simulink model "EPT"  (R2019b)
settings: Solver=FixedStepDiscrete  StartTime=0.0  StopTime=5  FixedStep=0.005  RelTol=1e-3  EnableMultiTasking=on
PreLoadFcn:
  | try, model_open; catch, disp('Error occurred while executing model pre-load callback: model_open.m'); disp('Please assure that the MATLAB working directory is set to the model directory before opening.'); end
InitFcn:
  | try, model_open; catch, end
undefined symbols (not defined in the file or in its folder): Bridge, GCM, H, ln, raptor_get_param_eval, raptor_get_safe_string, raptor_xcp_function
libraries: Raptor_lib x2810, simulink x374, hdlsllib x19
(part 42 of 45)

== system EPT/Foreground_TimeBase_5ms/E//W /BP-OBU_E//W/BP-OBU_E//W/BP-OBU_Warning//Fault_G5/Delay41/CycleTrigger ==
  In1 : Inport
  In2 : Inport  Port=2
  Add : Sum
  Add2 : Sum  Inputs=+-
  Constant2 : Constant  Value=0
  Constant3 : Constant
  Data Type Conversion1 : DataTypeConversion
  Data Type Conversion2 : DataTypeConversion
  Relational Operator1 : RelationalOperator  OutDataTypeStr=boolean  RndMeth=Simplest
  Saturation : Saturate  UpperLimit=inf  LowerLimit=2
  Switch : Switch  Threshold=1
  Unit Delay : UnitDelay  SampleTime=-1  HasFrameUpgradeWarning=on
  Trigger : Outport  VectorParamsAs1DForOutWhenUnconnected=off
  wires:
  Constant3/1 -> Add2/2
  In2/1 -> Saturation/1
  Add2/1 -> Data Type Conversion1/1
  Data Type Conversion2/1 -> Switch/2, Add/2
  Constant2/1 -> Switch/3
  Data Type Conversion1/1 -> Relational Operator1/2
  Relational Operator1/1 -> Trigger/1
  Switch/1 -> Unit Delay/1, Relational Operator1/1
  Unit Delay/1 -> Add/1
  In1/1 -> Data Type Conversion2/1
  Add/1 -> Switch/1
  Saturation/1 -> Add2/1

== system EPT/Foreground_TimeBase_5ms/E//W /BP-OBU_E//W/BP-OBU_E//W/BP-OBU_Warning//Fault_G5/Delay42/CycleTrigger ==
  In1 : Inport
  In2 : Inport  Port=2
  Add : Sum
  Add2 : Sum  Inputs=+-
  Constant2 : Constant  Value=0
  Constant3 : Constant
  Data Type Conversion1 : DataTypeConversion
  Data Type Conversion2 : DataTypeConversion
  Relational Operator1 : RelationalOperator  OutDataTypeStr=boolean  RndMeth=Simplest
  Saturation : Saturate  UpperLimit=inf  LowerLimit=2
  Switch : Switch  Threshold=1
  Unit Delay : UnitDelay  SampleTime=-1  HasFrameUpgradeWarning=on
  Trigger : Outport  VectorParamsAs1DForOutWhenUnconnected=off
  wires:
  Saturation/1 -> Add2/1
  Add/1 -> Switch/1
  In1/1 -> Data Type Conversion2/1
  Unit Delay/1 -> Add/1
  Switch/1 -> Relational Operator1/1, Unit Delay/1
  Relational Operator1/1 -> Trigger/1
  Data Type Conversion1/1 -> Relational Operator1/2
  Constant2/1 -> Switch/3
  Data Type Conversion2/1 -> Add/2, Switch/2
  Add2/1 -> Data Type Conversion1/1
  In2/1 -> Saturation/1
  Constant3/1 -> Add2/2

== system EPT/Foreground_TimeBase_5ms/E//W /BP-OBU_E//W/BP-OBU_E//W/BP-OBU_Warning//Fault_G5/Delay43/CycleTrigger ==
  In1 : Inport
  In2 : Inport  Port=2
  Add : Sum
  Add2 : Sum  Inputs=+-
  Constant2 : Constant  Value=0
  Constant3 : Constant
  Data Type Conversion1 : DataTypeConversion
  Data Type Conversion2 : DataTypeConversion
  Relational Operator1 : RelationalOperator  OutDataTypeStr=boolean  RndMeth=Simplest
  Saturation : Saturate  UpperLimit=inf  LowerLimit=2
  Switch : Switch  Threshold=1
  Unit Delay : UnitDelay  SampleTime=-1  HasFrameUpgradeWarning=on
  Trigger : Outport  VectorParamsAs1DForOutWhenUnconnected=off
  wires:
  Constant3/1 -> Add2/2
  In2/1 -> Saturation/1
  Add2/1 -> Data Type Conversion1/1
  Data Type Conversion2/1 -> Switch/2, Add/2
  Constant2/1 -> Switch/3
  Data Type Conversion1/1 -> Relational Operator1/2
  Relational Operator1/1 -> Trigger/1
  Switch/1 -> Unit Delay/1, Relational Operator1/1
  Unit Delay/1 -> Add/1
  In1/1 -> Data Type Conversion2/1
  Add/1 -> Switch/1
  Saturation/1 -> Add2/1

== system EPT/Foreground_TimeBase_5ms/E//W /BP-OBU_E//W/BP-OBU_E//W/BP-OBU_Warning//Fault_G5/Delay44/CycleTrigger ==
  In1 : Inport
  In2 : Inport  Port=2
  Add : Sum
  Add2 : Sum  Inputs=+-
  Constant2 : Constant  Value=0
  Constant3 : Constant
  Data Type Conversion1 : DataTypeConversion
  Data Type Conversion2 : DataTypeConversion
  Relational Operator1 : RelationalOperator  OutDataTypeStr=boolean  RndMeth=Simplest
  Saturation : Saturate  UpperLimit=inf  LowerLimit=2
  Switch : Switch  Threshold=1
  Unit Delay : UnitDelay  SampleTime=-1  HasFrameUpgradeWarning=on
  Trigger : Outport  VectorParamsAs1DForOutWhenUnconnected=off
  wires:
  Saturation/1 -> Add2/1
  Add/1 -> Switch/1
  In1/1 -> Data Type Conversion2/1
  Unit Delay/1 -> Add/1
  Switch/1 -> Relational Operator1/1, Unit Delay/1
  Relational Operator1/1 -> Trigger/1
  Data Type Conversion1/1 -> Relational Operator1/2
  Constant2/1 -> Switch/3
  Data Type Conversion2/1 -> Add/2, Switch/2
  Add2/1 -> Data Type Conversion1/1
  In2/1 -> Saturation/1
  Constant3/1 -> Add2/2

== system EPT/Foreground_TimeBase_5ms/E//W /CAN_E//W/CAN_Fault/BCU CAN Fault/BCU LifeCycle Fault/If Action Subsystem10 ==
  LifeCycle : Inport
  CanWork : Inport  Port=2
  Enable : EnablePort
  Add Constant : Bias  Bias=1
  Constant1 : Constant  Value=5
  Delay1 : Delay  DelayLength=1  InitialCondition=0
  Detect Change : simulink/Logic and Bit Operations/Detect Change  vinit=0  OutDataTypeStr=boolean
  Logical Operator : Logic  AllPortsSameDT=off  OutDataTypeStr=boolean
  NOT : Logic  Operator=NOT  IconShape=distinctive  AllPortsSameDT=off  OutDataTypeStr=boolean
  NOT1 : Logic  Operator=NOT  IconShape=distinctive  AllPortsSameDT=off  OutDataTypeStr=boolean
  Relational Operator : RelationalOperator  Operator=>  OutDataTypeStr=boolean  RndMeth=Simplest
  Switch1 : Switch  Criteria=u2 > Threshold
  Switch4 : Switch  Criteria=u2 > Threshold
  initTimeFlag : Subsystem
  Trigger : Outport  VectorParamsAs1DForOutWhenUnconnected=off
  wires:
  NOT/1 -> Logical Operator/1
  Constant1/1 -> Relational Operator/2
  CanWork/1 -> NOT1/1, Logical Operator/2
  Detect Change/1 -> NOT/1
  Delay1/1 -> Add Constant/1
  Logical Operator/1 -> Switch4/2
  Relational Operator/1 -> Trigger/1
  Add Constant/1 -> Switch4/1
  Switch4/1 -> Switch1/3
  Switch1/1 -> Delay1/1, Relational Operator/1
  LifeCycle/1 -> Detect Change/1
  NOT1/1 -> Switch1/2

== system EPT/Foreground_TimeBase_5ms/E//W /CAN_E//W/CAN_Fault/BCU CAN Fault/BCU LifeCycle Fault/If Action Subsystem11 ==
  LifeCycle : Inport
  CanWork : Inport  Port=2
  Enable : EnablePort
  Add Constant : Bias  Bias=1
  Constant1 : Constant  Value=5
  Delay1 : Delay  DelayLength=1  InitialCondition=0
  Detect Change : simulink/Logic and Bit Operations/Detect Change  vinit=0  OutDataTypeStr=boolean
  Logical Operator : Logic  AllPortsSameDT=off  OutDataTypeStr=boolean
  NOT : Logic  Operator=NOT  IconShape=distinctive  AllPortsSameDT=off  OutDataTypeStr=boolean
  NOT1 : Logic  Operator=NOT  IconShape=distinctive  AllPortsSameDT=off  OutDataTypeStr=boolean
  Relational Operator : RelationalOperator  Operator=>  OutDataTypeStr=boolean  RndMeth=Simplest
  Switch1 : Switch  Criteria=u2 > Threshold
  Switch4 : Switch  Criteria=u2 > Threshold
  initTimeFlag : Subsystem
  Trigger : Outport  VectorParamsAs1DForOutWhenUnconnected=off
  wires:
  NOT/1 -> Logical Operator/1
  Constant1/1 -> Relational Operator/2
  CanWork/1 -> NOT1/1, Logical Operator/2
  Detect Change/1 -> NOT/1
  Delay1/1 -> Add Constant/1
  Logical Operator/1 -> Switch4/2
  Relational Operator/1 -> Trigger/1
  Add Constant/1 -> Switch4/1
  Switch4/1 -> Switch1/3
  Switch1/1 -> Delay1/1, Relational Operator/1
  LifeCycle/1 -> Detect Change/1
  NOT1/1 -> Switch1/2

== system EPT/Foreground_TimeBase_5ms/E//W /CAN_E//W/CAN_Fault/BCU CAN Fault/BCU LifeCycle Fault/If Action Subsystem12 ==
  LifeCycle : Inport
  CanWork : Inport  Port=2
  Enable : EnablePort
  Add Constant : Bias  Bias=1
  Constant1 : Constant  Value=5
  Delay1 : Delay  DelayLength=1  InitialCondition=0
  Detect Change : simulink/Logic and Bit Operations/Detect Change  vinit=0  OutDataTypeStr=boolean
  Logical Operator : Logic  AllPortsSameDT=off  OutDataTypeStr=boolean
  NOT : Logic  Operator=NOT  IconShape=distinctive  AllPortsSameDT=off  OutDataTypeStr=boolean
  NOT1 : Logic  Operator=NOT  IconShape=distinctive  AllPortsSameDT=off  OutDataTypeStr=boolean
  Relational Operator : RelationalOperator  Operator=>  OutDataTypeStr=boolean  RndMeth=Simplest
  Switch1 : Switch  Criteria=u2 > Threshold
  Switch4 : Switch  Criteria=u2 > Threshold
  initTimeFlag : Subsystem
  Trigger : Outport  VectorParamsAs1DForOutWhenUnconnected=off
  wires:
  NOT/1 -> Logical Operator/1
  Constant1/1 -> Relational Operator/2
  CanWork/1 -> NOT1/1, Logical Operator/2
  Detect Change/1 -> NOT/1
  Delay1/1 -> Add Constant/1
  Logical Operator/1 -> Switch4/2
  Relational Operator/1 -> Trigger/1
  Add Constant/1 -> Switch4/1
  Switch4/1 -> Switch1/3
  Switch1/1 -> Delay1/1, Relational Operator/1
  LifeCycle/1 -> Detect Change/1
  NOT1/1 -> Switch1/2

== system EPT/Foreground_TimeBase_5ms/E//W /CAN_E//W/CAN_Fault/BCU CAN Fault/BCU LifeCycle Fault/If Action Subsystem13 ==
  LifeCycle : Inport
  CanWork : Inport  Port=2
  Enable : EnablePort
  Add Constant : Bias  Bias=1
  Constant1 : Constant  Value=5
  Delay1 : Delay  DelayLength=1  InitialCondition=0
  Detect Change : simulink/Logic and Bit Operations/Detect Change  vinit=0  OutDataTypeStr=boolean
  Logical Operator : Logic  AllPortsSameDT=off  OutDataTypeStr=boolean
  NOT : Logic  Operator=NOT  IconShape=distinctive  AllPortsSameDT=off  OutDataTypeStr=boolean
  NOT1 : Logic  Operator=NOT  IconShape=distinctive  AllPortsSameDT=off  OutDataTypeStr=boolean
  Relational Operator : RelationalOperator  Operator=>  OutDataTypeStr=boolean  RndMeth=Simplest
  Switch1 : Switch  Criteria=u2 > Threshold
  Switch4 : Switch  Criteria=u2 > Threshold
  initTimeFlag : Subsystem
  Trigger : Outport  VectorParamsAs1DForOutWhenUnconnected=off
  wires:
  NOT1/1 -> Switch1/2
  LifeCycle/1 -> Detect Change/1
  Switch1/1 -> Relational Operator/1, Delay1/1
  Switch4/1 -> Switch1/3
  Add Constant/1 -> Switch4/1
  Relational Operator/1 -> Trigger/1
  Logical Operator/1 -> Switch4/2
  Delay1/1 -> Add Constant/1
  Detect Change/1 -> NOT/1
  CanWork/1 -> Logical Operator/2, NOT1/1
  Constant1/1 -> Relational Operator/2
  NOT/1 -> Logical Operator/1

== system EPT/Foreground_TimeBase_5ms/E//W /CAN_E//W/CAN_Fault/BCU CAN Fault/BCU LifeCycle Fault/If Action Subsystem18 ==
  LifeCycle : Inport
  CanWork : Inport  Port=2
  Enable : EnablePort
  Add Constant : Bias  Bias=1
  Constant1 : Constant  Value=5
  Delay1 : Delay  DelayLength=1  InitialCondition=0
  Detect Change : simulink/Logic and Bit Operations/Detect Change  vinit=0  OutDataTypeStr=boolean
  Logical Operator : Logic  AllPortsSameDT=off  OutDataTypeStr=boolean
  NOT : Logic  Operator=NOT  IconShape=distinctive  AllPortsSameDT=off  OutDataTypeStr=boolean
  NOT1 : Logic  Operator=NOT  IconShape=distinctive  AllPortsSameDT=off  OutDataTypeStr=boolean
  Relational Operator : RelationalOperator  Operator=>  OutDataTypeStr=boolean  RndMeth=Simplest
  Switch1 : Switch  Criteria=u2 > Threshold
  Switch4 : Switch  Criteria=u2 > Threshold
  initTimeFlag : Subsystem
  Trigger : Outport  VectorParamsAs1DForOutWhenUnconnected=off
  wires:
  NOT1/1 -> Switch1/2
  LifeCycle/1 -> Detect Change/1
  Switch1/1 -> Relational Operator/1, Delay1/1
  Switch4/1 -> Switch1/3
  Add Constant/1 -> Switch4/1
  Relational Operator/1 -> Trigger/1
  Logical Operator/1 -> Switch4/2
  Delay1/1 -> Add Constant/1
  Detect Change/1 -> NOT/1
  CanWork/1 -> Logical Operator/2, NOT1/1
  Constant1/1 -> Relational Operator/2
  NOT/1 -> Logical Operator/1

== system EPT/Foreground_TimeBase_5ms/E//W /CAN_E//W/CAN_Fault/BCU CAN Fault/BCU LifeCycle Fault/If Action Subsystem9 ==
  LifeCycle : Inport
  CanWork : Inport  Port=2
  Enable : EnablePort
  Add Constant : Bias  Bias=1
  Constant1 : Constant  Value=5
  Delay1 : Delay  DelayLength=1  InitialCondition=0
  Detect Change : simulink/Logic and Bit Operations/Detect Change  vinit=0  OutDataTypeStr=boolean
  Logical Operator : Logic  AllPortsSameDT=off  OutDataTypeStr=boolean
  NOT : Logic  Operator=NOT  IconShape=distinctive  AllPortsSameDT=off  OutDataTypeStr=boolean
  NOT1 : Logic  Operator=NOT  IconShape=distinctive  AllPortsSameDT=off  OutDataTypeStr=boolean
  Relational Operator : RelationalOperator  Operator=>  OutDataTypeStr=boolean  RndMeth=Simplest
  Switch1 : Switch  Criteria=u2 > Threshold
  Switch4 : Switch  Criteria=u2 > Threshold
  initTimeFlag : Subsystem
  Trigger : Outport  VectorParamsAs1DForOutWhenUnconnected=off
  wires:
  NOT/1 -> Logical Operator/1
  Constant1/1 -> Relational Operator/2
  CanWork/1 -> NOT1/1, Logical Operator/2
  Detect Change/1 -> NOT/1
  Delay1/1 -> Add Constant/1
  Logical Operator/1 -> Switch4/2
  Relational Operator/1 -> Trigger/1
  Add Constant/1 -> Switch4/1
  Switch4/1 -> Switch1/3
  Switch1/1 -> Delay1/1, Relational Operator/1
  LifeCycle/1 -> Detect Change/1
  NOT1/1 -> Switch1/2

== system EPT/Foreground_TimeBase_5ms/E//W /CAN_E//W/CAN_Fault/BCU CAN Fault/BCU LifeCycle Fault/Latch10 ==
  Latch : Inport
  Reset : Inport  Port=2
  Switch1 : Switch  Criteria=u2 > Threshold
  Switch3 : Switch  Criteria=u2 > Threshold
  Unit Delay1 : UnitDelay  SampleTime=-1  HasFrameUpgradeWarning=on
  Output : Outport  VectorParamsAs1DForOutWhenUnconnected=off
  wires:
  Switch1/1 -> Switch3/3
  Latch/1 -> Switch1/2, Switch1/1
  Reset/1 -> Switch3/2
  Switch3/1 -> Unit Delay1/1, Output/1
  Unit Delay1/1 -> Switch1/3

== system EPT/Foreground_TimeBase_5ms/E//W /CAN_E//W/CAN_Fault/BCU CAN Fault/BCU LifeCycle Fault/Latch11 ==
  Latch : Inport
  Reset : Inport  Port=2
  Switch1 : Switch  Criteria=u2 > Threshold
  Switch3 : Switch  Criteria=u2 > Threshold
  Unit Delay1 : UnitDelay  SampleTime=-1  HasFrameUpgradeWarning=on
  Output : Outport  VectorParamsAs1DForOutWhenUnconnected=off
  wires:
  Switch1/1 -> Switch3/3
  Latch/1 -> Switch1/2, Switch1/1
  Reset/1 -> Switch3/2
  Switch3/1 -> Unit Delay1/1, Output/1
  Unit Delay1/1 -> Switch1/3

== system EPT/Foreground_TimeBase_5ms/E//W /CAN_E//W/CAN_Fault/BCU CAN Fault/BCU LifeCycle Fault/Latch12 ==
  Latch : Inport
  Reset : Inport  Port=2
  Switch1 : Switch  Criteria=u2 > Threshold
  Switch3 : Switch  Criteria=u2 > Threshold
  Unit Delay1 : UnitDelay  SampleTime=-1  HasFrameUpgradeWarning=on
  Output : Outport  VectorParamsAs1DForOutWhenUnconnected=off
  wires:
  Switch1/1 -> Switch3/3
  Latch/1 -> Switch1/2, Switch1/1
  Reset/1 -> Switch3/2
  Switch3/1 -> Unit Delay1/1, Output/1
  Unit Delay1/1 -> Switch1/3

== system EPT/Foreground_TimeBase_5ms/E//W /CAN_E//W/CAN_Fault/BCU CAN Fault/BCU LifeCycle Fault/Latch13 ==
  Latch : Inport
  Reset : Inport  Port=2
  Switch1 : Switch  Criteria=u2 > Threshold
  Switch3 : Switch  Criteria=u2 > Threshold
  Unit Delay1 : UnitDelay  SampleTime=-1  HasFrameUpgradeWarning=on
  Output : Outport  VectorParamsAs1DForOutWhenUnconnected=off
  wires:
  Switch1/1 -> Switch3/3
  Latch/1 -> Switch1/2, Switch1/1
  Reset/1 -> Switch3/2
  Switch3/1 -> Unit Delay1/1, Output/1
  Unit Delay1/1 -> Switch1/3

== system EPT/Foreground_TimeBase_5ms/E//W /CAN_E//W/CAN_Fault/BCU CAN Fault/BCU LifeCycle Fault/Latch14 ==
  Latch : Inport
  Reset : Inport  Port=2
  Switch1 : Switch  Criteria=u2 > Threshold
  Switch3 : Switch  Criteria=u2 > Threshold
  Unit Delay1 : UnitDelay  SampleTime=-1  HasFrameUpgradeWarning=on
  Output : Outport  VectorParamsAs1DForOutWhenUnconnected=off
  wires:
  Unit Delay1/1 -> Switch1/3
  Switch3/1 -> Output/1, Unit Delay1/1
  Reset/1 -> Switch3/2
  Latch/1 -> Switch1/1, Switch1/2
  Switch1/1 -> Switch3/3

== system EPT/Foreground_TimeBase_5ms/E//W /CAN_E//W/CAN_Fault/BCU CAN Fault/BCU LifeCycle Fault/Latch19 ==
  Latch : Inport
  Reset : Inport  Port=2
  Switch1 : Switch  Criteria=u2 > Threshold
  Switch3 : Switch  Criteria=u2 > Threshold
  Unit Delay1 : UnitDelay  SampleTime=-1  HasFrameUpgradeWarning=on
  Output : Outport  VectorParamsAs1DForOutWhenUnconnected=off
  wires:
  Unit Delay1/1 -> Switch1/3
  Switch3/1 -> Output/1, Unit Delay1/1
  Reset/1 -> Switch3/2
  Latch/1 -> Switch1/1, Switch1/2
  Switch1/1 -> Switch3/3

== system EPT/Foreground_TimeBase_5ms/E//W /CAN_E//W/CAN_Fault/BCU CAN Fault/deBounce 12/CycleTrigger1 ==
  In1 : Inport
  In2 : Inport  Port=2
  Add : Sum
  Add1 : Sum
  Add2 : Sum  Inputs=+-
  Constant1 : Constant
  Constant2 : Constant  Value=0
  Constant3 : Constant
  Data Type Conversion1 : DataTypeConversion
  Data Type Conversion2 : DataTypeConversion
  Display : Display
  Relational Operator1 : RelationalOperator  OutDataTypeStr=boolean  RndMeth=Simplest
  Saturation : Saturate  UpperLimit=inf  LowerLimit=2
  Scope : Scope
  Scope1 : Scope
  Scope2 : Scope
  Switch : Switch  Threshold=1
  Unit Delay : UnitDelay  SampleTime=-1  HasFrameUpgradeWarning=on
  Unit Delay1 : UnitDelay  SampleTime=-1  HasFrameUpgradeWarning=on
  Trigger : Outport  VectorParamsAs1DForOutWhenUnconnected=off
  wires:
  Constant3/1 -> Add2/2
  In2/1 -> Saturation/1
  Add2/1 -> Data Type Conversion1/1
  Data Type Conversion2/1 -> Switch/2, Add/2
  Constant2/1 -> Switch/3
  Data Type Conversion1/1 -> Relational Operator1/2
  Relational Operator1/1 -> Trigger/1, Scope2/1
  Constant1/1 -> Add1/2
  Unit Delay1/1 -> Add1/1
  Add1/1 -> Display/1, Unit Delay1/1, Scope/1
  Switch/1 -> Unit Delay/1, Scope1/1, Relational Operator1/1
  Unit Delay/1 -> Add/1
  In1/1 -> Data Type Conversion2/1
  Add/1 -> Switch/1
  Saturation/1 -> Add2/1

== system EPT/Foreground_TimeBase_5ms/E//W /CAN_E//W/CAN_Fault/BCU CAN Fault/deBounce 13/CycleTrigger1 ==
  In1 : Inport
  In2 : Inport  Port=2
  Add : Sum
  Add1 : Sum
  Add2 : Sum  Inputs=+-
  Constant1 : Constant
  Constant2 : Constant  Value=0
  Constant3 : Constant
  Data Type Conversion1 : DataTypeConversion
  Data Type Conversion2 : DataTypeConversion
  Display : Display
  Relational Operator1 : RelationalOperator  OutDataTypeStr=boolean  RndMeth=Simplest
  Saturation : Saturate  UpperLimit=inf  LowerLimit=2
  Scope : Scope
  Scope1 : Scope
  Scope2 : Scope
  Switch : Switch  Threshold=1
  Unit Delay : UnitDelay  SampleTime=-1  HasFrameUpgradeWarning=on
  Unit Delay1 : UnitDelay  SampleTime=-1  HasFrameUpgradeWarning=on
  Trigger : Outport  VectorParamsAs1DForOutWhenUnconnected=off
  wires:
  Saturation/1 -> Add2/1
  Add/1 -> Switch/1
  In1/1 -> Data Type Conversion2/1
  Unit Delay/1 -> Add/1
  Switch/1 -> Relational Operator1/1, Scope1/1, Unit Delay/1
  Add1/1 -> Scope/1, Unit Delay1/1, Display/1
  Unit Delay1/1 -> Add1/1
  Constant1/1 -> Add1/2
  Relational Operator1/1 -> Scope2/1, Trigger/1
  Data Type Conversion1/1 -> Relational Operator1/2
  Constant2/1 -> Switch/3
  Data Type Conversion2/1 -> Add/2, Switch/2
  Add2/1 -> Data Type Conversion1/1
  In2/1 -> Saturation/1
  Constant3/1 -> Add2/2

== system EPT/Foreground_TimeBase_5ms/E//W /CAN_E//W/CAN_Fault/BCU CAN Fault/deBounce 14/CycleTrigger1 ==
  In1 : Inport
  In2 : Inport  Port=2
  Add : Sum
  Add1 : Sum
  Add2 : Sum  Inputs=+-
  Constant1 : Constant
  Constant2 : Constant  Value=0
  Constant3 : Constant
  Data Type Conversion1 : DataTypeConversion
  Data Type Conversion2 : DataTypeConversion
  Display : Display
  Relational Operator1 : RelationalOperator  OutDataTypeStr=boolean  RndMeth=Simplest
  Saturation : Saturate  UpperLimit=inf  LowerLimit=2
  Scope : Scope
  Scope1 : Scope
  Scope2 : Scope
  Switch : Switch  Threshold=1
  Unit Delay : UnitDelay  SampleTime=-1  HasFrameUpgradeWarning=on
  Unit Delay1 : UnitDelay  SampleTime=-1  HasFrameUpgradeWarning=on
  Trigger : Outport  VectorParamsAs1DForOutWhenUnconnected=off
  wires:
  Constant3/1 -> Add2/2
  In2/1 -> Saturation/1
  Add2/1 -> Data Type Conversion1/1
  Data Type Conversion2/1 -> Switch/2, Add/2
  Constant2/1 -> Switch/3
  Data Type Conversion1/1 -> Relational Operator1/2
  Relational Operator1/1 -> Trigger/1, Scope2/1
  Constant1/1 -> Add1/2
  Unit Delay1/1 -> Add1/1
  Add1/1 -> Display/1, Unit Delay1/1, Scope/1
  Switch/1 -> Unit Delay/1, Scope1/1, Relational Operator1/1
  Unit Delay/1 -> Add/1
  In1/1 -> Data Type Conversion2/1
  Add/1 -> Switch/1
  Saturation/1 -> Add2/1

== system EPT/Foreground_TimeBase_5ms/E//W /CAN_E//W/CAN_Fault/BCU CAN Fault/deBounce 15/CycleTrigger1 ==
  In1 : Inport
  In2 : Inport  Port=2
  Add : Sum
  Add1 : Sum
  Add2 : Sum  Inputs=+-
  Constant1 : Constant
  Constant2 : Constant  Value=0
  Constant3 : Constant
  Data Type Conversion1 : DataTypeConversion
  Data Type Conversion2 : DataTypeConversion
  Display : Display
  Relational Operator1 : RelationalOperator  OutDataTypeStr=boolean  RndMeth=Simplest
  Saturation : Saturate  UpperLimit=inf  LowerLimit=2
  Scope : Scope
  Scope1 : Scope
  Scope2 : Scope
  Switch : Switch  Threshold=1
  Unit Delay : UnitDelay  SampleTime=-1  HasFrameUpgradeWarning=on
  Unit Delay1 : UnitDelay  SampleTime=-1  HasFrameUpgradeWarning=on
  Trigger : Outport  VectorParamsAs1DForOutWhenUnconnected=off
  wires:
  Saturation/1 -> Add2/1
  Add/1 -> Switch/1
  In1/1 -> Data Type Conversion2/1
  Unit Delay/1 -> Add/1
  Switch/1 -> Relational Operator1/1, Scope1/1, Unit Delay/1
  Add1/1 -> Scope/1, Unit Delay1/1, Display/1
  Unit Delay1/1 -> Add1/1
  Constant1/1 -> Add1/2
  Relational Operator1/1 -> Scope2/1, Trigger/1
  Data Type Conversion1/1 -> Relational Operator1/2
  Constant2/1 -> Switch/3
  Data Type Conversion2/1 -> Add/2, Switch/2
  Add2/1 -> Data Type Conversion1/1
  In2/1 -> Saturation/1
  Constant3/1 -> Add2/2

== system EPT/Foreground_TimeBase_5ms/E//W /CAN_E//W/CAN_Fault/BCU CAN Fault/deBounce 16/CycleTrigger1 ==
  In1 : Inport
  In2 : Inport  Port=2
  Add : Sum
  Add1 : Sum
  Add2 : Sum  Inputs=+-
  Constant1 : Constant
  Constant2 : Constant  Value=0
  Constant3 : Constant
  Data Type Conversion1 : DataTypeConversion
  Data Type Conversion2 : DataTypeConversion
  Display : Display
  Relational Operator1 : RelationalOperator  OutDataTypeStr=boolean  RndMeth=Simplest
  Saturation : Saturate  UpperLimit=inf  LowerLimit=2
  Scope : Scope
  Scope1 : Scope
  Scope2 : Scope
  Switch : Switch  Threshold=1
  Unit Delay : UnitDelay  SampleTime=-1  HasFrameUpgradeWarning=on
  Unit Delay1 : UnitDelay  SampleTime=-1  HasFrameUpgradeWarning=on
  Trigger : Outport  VectorParamsAs1DForOutWhenUnconnected=off
  wires:
  Constant3/1 -> Add2/2
  In2/1 -> Saturation/1
  Add2/1 -> Data Type Conversion1/1
  Data Type Conversion2/1 -> Switch/2, Add/2
  Constant2/1 -> Switch/3
  Data Type Conversion1/1 -> Relational Operator1/2
  Relational Operator1/1 -> Trigger/1, Scope2/1
  Constant1/1 -> Add1/2
  Unit Delay1/1 -> Add1/1
  Add1/1 -> Display/1, Unit Delay1/1, Scope/1
  Switch/1 -> Unit Delay/1, Scope1/1, Relational Operator1/1
  Unit Delay/1 -> Add/1
  In1/1 -> Data Type Conversion2/1
  Add/1 -> Switch/1
  Saturation/1 -> Add2/1

== system EPT/Foreground_TimeBase_5ms/E//W /CAN_E//W/CAN_Fault/BCU CAN Fault/deBounce 4/CycleTrigger1 ==
  In1 : Inport
  In2 : Inport  Port=2
  Add : Sum
  Add1 : Sum
  Add2 : Sum  Inputs=+-
  Constant1 : Constant
  Constant2 : Constant  Value=0
  Constant3 : Constant
  Data Type Conversion1 : DataTypeConversion
  Data Type Conversion2 : DataTypeConversion
  Display : Display
  Relational Operator1 : RelationalOperator  OutDataTypeStr=boolean  RndMeth=Simplest
  Saturation : Saturate  UpperLimit=inf  LowerLimit=2
  Scope : Scope
  Scope1 : Scope
  Scope2 : Scope
  Switch : Switch  Threshold=1
  Unit Delay : UnitDelay  SampleTime=-1  HasFrameUpgradeWarning=on
  Unit Delay1 : UnitDelay  SampleTime=-1  HasFrameUpgradeWarning=on
  Trigger : Outport  VectorParamsAs1DForOutWhenUnconnected=off
  wires:
  Saturation/1 -> Add2/1
  Add/1 -> Switch/1
  In1/1 -> Data Type Conversion2/1
  Unit Delay/1 -> Add/1
  Switch/1 -> Relational Operator1/1, Scope1/1, Unit Delay/1
  Add1/1 -> Scope/1, Unit Delay1/1, Display/1
  Unit Delay1/1 -> Add1/1
  Constant1/1 -> Add1/2
  Relational Operator1/1 -> Scope2/1, Trigger/1
  Data Type Conversion1/1 -> Relational Operator1/2
  Constant2/1 -> Switch/3
  Data Type Conversion2/1 -> Add/2, Switch/2
  Add2/1 -> Data Type Conversion1/1
  In2/1 -> Saturation/1
  Constant3/1 -> Add2/2

== system EPT/Foreground_TimeBase_5ms/E//W /CAN_E//W/CAN_Fault/BCU CAN Fault/deBounce 5/CycleTrigger1 ==
  In1 : Inport
  In2 : Inport  Port=2
  Add : Sum
  Add1 : Sum
  Add2 : Sum  Inputs=+-
  Constant1 : Constant
  Constant2 : Constant  Value=0
  Constant3 : Constant
  Data Type Conversion1 : DataTypeConversion
  Data Type Conversion2 : DataTypeConversion
  Display : Display
  Relational Operator1 : RelationalOperator  OutDataTypeStr=boolean  RndMeth=Simplest
  Saturation : Saturate  UpperLimit=inf  LowerLimit=2
  Scope : Scope
  Scope1 : Scope
  Scope2 : Scope
  Switch : Switch  Threshold=1
  Unit Delay : UnitDelay  SampleTime=-1  HasFrameUpgradeWarning=on
  Unit Delay1 : UnitDelay  SampleTime=-1  HasFrameUpgradeWarning=on
  Trigger : Outport  VectorParamsAs1DForOutWhenUnconnected=off
  wires:
  Constant3/1 -> Add2/2
  In2/1 -> Saturation/1
  Add2/1 -> Data Type Conversion1/1
  Data Type Conversion2/1 -> Switch/2, Add/2
  Constant2/1 -> Switch/3
  Data Type Conversion1/1 -> Relational Operator1/2
  Relational Operator1/1 -> Trigger/1, Scope2/1
  Constant1/1 -> Add1/2
  Unit Delay1/1 -> Add1/1
  Add1/1 -> Display/1, Unit Delay1/1, Scope/1
  Switch/1 -> Unit Delay/1, Scope1/1, Relational Operator1/1
  Unit Delay/1 -> Add/1
  In1/1 -> Data Type Conversion2/1
  Add/1 -> Switch/1
  Saturation/1 -> Add2/1

== system EPT/Foreground_TimeBase_5ms/E//W /CAN_E//W/CAN_Fault/BCU CAN Fault/deBounce 6/CycleTrigger1 ==
  In1 : Inport
  In2 : Inport  Port=2
  Add : Sum
  Add1 : Sum
  Add2 : Sum  Inputs=+-
  Constant1 : Constant
  Constant2 : Constant  Value=0
  Constant3 : Constant
  Data Type Conversion1 : DataTypeConversion
  Data Type Conversion2 : DataTypeConversion
  Display : Display
  Relational Operator1 : RelationalOperator  OutDataTypeStr=boolean  RndMeth=Simplest
  Saturation : Saturate  UpperLimit=inf  LowerLimit=2
  Scope : Scope
  Scope1 : Scope
  Scope2 : Scope
  Switch : Switch  Threshold=1
  Unit Delay : UnitDelay  SampleTime=-1  HasFrameUpgradeWarning=on
  Unit Delay1 : UnitDelay  SampleTime=-1  HasFrameUpgradeWarning=on
  Trigger : Outport  VectorParamsAs1DForOutWhenUnconnected=off
  wires:
  Saturation/1 -> Add2/1
  Add/1 -> Switch/1
  In1/1 -> Data Type Conversion2/1
  Unit Delay/1 -> Add/1
  Switch/1 -> Relational Operator1/1, Scope1/1, Unit Delay/1
  Add1/1 -> Scope/1, Unit Delay1/1, Display/1
  Unit Delay1/1 -> Add1/1
  Constant1/1 -> Add1/2
  Relational Operator1/1 -> Scope2/1, Trigger/1
  Data Type Conversion1/1 -> Relational Operator1/2
  Constant2/1 -> Switch/3
  Data Type Conversion2/1 -> Add/2, Switch/2
  Add2/1 -> Data Type Conversion1/1
  In2/1 -> Saturation/1
  Constant3/1 -> Add2/2

== system EPT/Foreground_TimeBase_5ms/E//W /CAN_E//W/CAN_Fault/BCU CAN Fault/deBounce 7/CycleTrigger1 ==
  In1 : Inport
  In2 : Inport  Port=2
  Add : Sum
  Add1 : Sum
  Add2 : Sum  Inputs=+-
  Constant1 : Constant
  Constant2 : Constant  Value=0
  Constant3 : Constant
  Data Type Conversion1 : DataTypeConversion
  Data Type Conversion2 : DataTypeConversion
  Display : Display
  Relational Operator1 : RelationalOperator  OutDataTypeStr=boolean  RndMeth=Simplest
  Saturation : Saturate  UpperLimit=inf  LowerLimit=2
  Scope : Scope
  Scope1 : Scope
  Scope2 : Scope
  Switch : Switch  Threshold=1
  Unit Delay : UnitDelay  SampleTime=-1  HasFrameUpgradeWarning=on
  Unit Delay1 : UnitDelay  SampleTime=-1  HasFrameUpgradeWarning=on
  Trigger : Outport  VectorParamsAs1DForOutWhenUnconnected=off
  wires:
  Constant3/1 -> Add2/2
  In2/1 -> Saturation/1
  Add2/1 -> Data Type Conversion1/1
  Data Type Conversion2/1 -> Switch/2, Add/2
  Constant2/1 -> Switch/3
  Data Type Conversion1/1 -> Relational Operator1/2
  Relational Operator1/1 -> Trigger/1, Scope2/1
  Constant1/1 -> Add1/2
  Unit Delay1/1 -> Add1/1
  Add1/1 -> Display/1, Unit Delay1/1, Scope/1
  Switch/1 -> Unit Delay/1, Scope1/1, Relational Operator1/1
  Unit Delay/1 -> Add/1
  In1/1 -> Data Type Conversion2/1
  Add/1 -> Switch/1
  Saturation/1 -> Add2/1

== system EPT/Foreground_TimeBase_5ms/E//W /CAN_E//W/CAN_Fault/BCU CAN Fault/deBounce 8/CycleTrigger1 ==
  In1 : Inport
  In2 : Inport  Port=2
  Add : Sum
  Add1 : Sum
  Add2 : Sum  Inputs=+-
  Constant1 : Constant
  Constant2 : Constant  Value=0
  Constant3 : Constant
  Data Type Conversion1 : DataTypeConversion
  Data Type Conversion2 : DataTypeConversion
  Display : Display
  Relational Operator1 : RelationalOperator  OutDataTypeStr=boolean  RndMeth=Simplest
  Saturation : Saturate  UpperLimit=inf  LowerLimit=2
  Scope : Scope
  Scope1 : Scope
  Scope2 : Scope
  Switch : Switch  Threshold=1
  Unit Delay : UnitDelay  SampleTime=-1  HasFrameUpgradeWarning=on
  Unit Delay1 : UnitDelay  SampleTime=-1  HasFrameUpgradeWarning=on
  Trigger : Outport  VectorParamsAs1DForOutWhenUnconnected=off
  wires:
  Saturation/1 -> Add2/1
  Add/1 -> Switch/1
  In1/1 -> Data Type Conversion2/1
  Unit Delay/1 -> Add/1
  Switch/1 -> Relational Operator1/1, Scope1/1, Unit Delay/1
  Add1/1 -> Scope/1, Unit Delay1/1, Display/1
  Unit Delay1/1 -> Add1/1
  Constant1/1 -> Add1/2
  Relational Operator1/1 -> Scope2/1, Trigger/1
  Data Type Conversion1/1 -> Relational Operator1/2
  Constant2/1 -> Switch/3
  Data Type Conversion2/1 -> Add/2, Switch/2
  Add2/1 -> Data Type Conversion1/1
  In2/1 -> Saturation/1
  Constant3/1 -> Add2/2

== system EPT/Foreground_TimeBase_5ms/E//W /CAN_E//W/CAN_Fault/BCU CAN Fault/deBounce 9/CycleTrigger1 ==
  In1 : Inport
  In2 : Inport  Port=2
  Add : Sum
  Add1 : Sum
  Add2 : Sum  Inputs=+-
  Constant1 : Constant
  Constant2 : Constant  Value=0
  Constant3 : Constant
  Data Type Conversion1 : DataTypeConversion
  Data Type Conversion2 : DataTypeConversion
  Display : Display
  Relational Operator1 : RelationalOperator  OutDataTypeStr=boolean  RndMeth=Simplest
  Saturation : Saturate  UpperLimit=inf  LowerLimit=2
  Scope : Scope
  Scope1 : Scope
  Scope2 : Scope
  Switch : Switch  Threshold=1
  Unit Delay : UnitDelay  SampleTime=-1  HasFrameUpgradeWarning=on
  Unit Delay1 : UnitDelay  SampleTime=-1  HasFrameUpgradeWarning=on
  Trigger : Outport  VectorParamsAs1DForOutWhenUnconnected=off
  wires:
  Constant3/1 -> Add2/2
  In2/1 -> Saturation/1
  Add2/1 -> Data Type Conversion1/1
  Data Type Conversion2/1 -> Switch/2, Add/2
  Constant2/1 -> Switch/3
  Data Type Conversion1/1 -> Relational Operator1/2
  Relational Operator1/1 -> Trigger/1, Scope2/1
  Constant1/1 -> Add1/2
  Unit Delay1/1 -> Add1/1
  Add1/1 -> Display/1, Unit Delay1/1, Scope/1
  Switch/1 -> Unit Delay/1, Scope1/1, Relational Operator1/1
  Unit Delay/1 -> Add/1
  In1/1 -> Data Type Conversion2/1
  Add/1 -> Switch/1
  Saturation/1 -> Add2/1

== system EPT/Foreground_TimeBase_5ms/E//W /CAN_E//W/CAN_Fault/DCDC CAN Fault/deBounce 1/CycleTrigger1 ==
  In1 : Inport
  In2 : Inport  Port=2
  Add : Sum
  Add1 : Sum
  Add2 : Sum  Inputs=+-
  Constant1 : Constant
  Constant2 : Constant  Value=0
  Constant3 : Constant
  Data Type Conversion1 : DataTypeConversion
  Data Type Conversion2 : DataTypeConversion
  Display : Display
  Relational Operator1 : RelationalOperator  OutDataTypeStr=boolean  RndMeth=Simplest
  Saturation : Saturate  UpperLimit=inf  LowerLimit=2
  Scope : Scope
  Scope1 : Scope
  Scope2 : Scope
  Switch : Switch  Threshold=1
  Unit Delay : UnitDelay  SampleTime=-1  HasFrameUpgradeWarning=on
  Unit Delay1 : UnitDelay  SampleTime=-1  HasFrameUpgradeWarning=on
  Trigger : Outport  VectorParamsAs1DForOutWhenUnconnected=off
  wires:
  Saturation/1 -> Add2/1
  Add/1 -> Switch/1
  In1/1 -> Data Type Conversion2/1
  Unit Delay/1 -> Add/1
  Switch/1 -> Relational Operator1/1, Scope1/1, Unit Delay/1
  Add1/1 -> Scope/1, Unit Delay1/1, Display/1
  Unit Delay1/1 -> Add1/1
  Constant1/1 -> Add1/2
  Relational Operator1/1 -> Scope2/1, Trigger/1
  Data Type Conversion1/1 -> Relational Operator1/2
  Constant2/1 -> Switch/3
  Data Type Conversion2/1 -> Add/2, Switch/2
  Add2/1 -> Data Type Conversion1/1
  In2/1 -> Saturation/1
  Constant3/1 -> Add2/2

== system EPT/Foreground_TimeBase_5ms/E//W /CAN_E//W/CAN_Fault/DCDC CAN Fault/deBounce 10/CycleTrigger1 ==
  In1 : Inport
  In2 : Inport  Port=2
  Add : Sum
  Add1 : Sum
  Add2 : Sum  Inputs=+-
  Constant1 : Constant
  Constant2 : Constant  Value=0
  Constant3 : Constant
  Data Type Conversion1 : DataTypeConversion
  Data Type Conversion2 : DataTypeConversion
  Display : Display
  Relational Operator1 : RelationalOperator  OutDataTypeStr=boolean  RndMeth=Simplest
  Saturation : Saturate  UpperLimit=inf  LowerLimit=2
  Scope : Scope
  Scope1 : Scope
  Scope2 : Scope
  Switch : Switch  Threshold=1
  Unit Delay : UnitDelay  SampleTime=-1  HasFrameUpgradeWarning=on
  Unit Delay1 : UnitDelay  SampleTime=-1  HasFrameUpgradeWarning=on
  Trigger : Outport  VectorParamsAs1DForOutWhenUnconnected=off
  wires:
  Constant3/1 -> Add2/2
  In2/1 -> Saturation/1
  Add2/1 -> Data Type Conversion1/1
  Data Type Conversion2/1 -> Switch/2, Add/2
  Constant2/1 -> Switch/3
  Data Type Conversion1/1 -> Relational Operator1/2
  Relational Operator1/1 -> Trigger/1, Scope2/1
  Constant1/1 -> Add1/2
  Unit Delay1/1 -> Add1/1
  Add1/1 -> Display/1, Unit Delay1/1, Scope/1
  Switch/1 -> Unit Delay/1, Scope1/1, Relational Operator1/1
  Unit Delay/1 -> Add/1
  In1/1 -> Data Type Conversion2/1
  Add/1 -> Switch/1
  Saturation/1 -> Add2/1

== system EPT/Foreground_TimeBase_5ms/E//W /CAN_E//W/CAN_Fault/ECHS CAN Fault/deBounce /CycleTrigger1 ==
  In1 : Inport
  In2 : Inport  Port=2
  Add : Sum
  Add1 : Sum
  Add2 : Sum  Inputs=+-
  Constant1 : Constant
  Constant2 : Constant  Value=0
  Constant3 : Constant
  Data Type Conversion1 : DataTypeConversion
  Data Type Conversion2 : DataTypeConversion
  Display : Display
  Relational Operator1 : RelationalOperator  OutDataTypeStr=boolean  RndMeth=Simplest
  Saturation : Saturate  UpperLimit=inf  LowerLimit=2
  Scope : Scope
  Scope1 : Scope
  Scope2 : Scope
  Switch : Switch  Threshold=1
  Unit Delay : UnitDelay  SampleTime=-1  HasFrameUpgradeWarning=on
  Unit Delay1 : UnitDelay  SampleTime=-1  HasFrameUpgradeWarning=on
  Trigger : Outport  VectorParamsAs1DForOutWhenUnconnected=off
  wires:
  Constant3/1 -> Add2/2
  In2/1 -> Saturation/1
  Add2/1 -> Data Type Conversion1/1
  Data Type Conversion2/1 -> Switch/2, Add/2
  Constant2/1 -> Switch/3
  Data Type Conversion1/1 -> Relational Operator1/2
  Relational Operator1/1 -> Trigger/1, Scope2/1
  Constant1/1 -> Add1/2
  Unit Delay1/1 -> Add1/1
  Add1/1 -> Display/1, Unit Delay1/1, Scope/1
  Switch/1 -> Unit Delay/1, Scope1/1, Relational Operator1/1
  Unit Delay/1 -> Add/1
  In1/1 -> Data Type Conversion2/1
  Add/1 -> Switch/1
  Saturation/1 -> Add2/1

== system EPT/Foreground_TimeBase_5ms/E//W /CAN_E//W/CAN_Fault/ECHS CAN Fault/deBounce 1/CycleTrigger1 ==
  In1 : Inport
  In2 : Inport  Port=2
  Add : Sum
  Add1 : Sum
  Add2 : Sum  Inputs=+-
  Constant1 : Constant
  Constant2 : Constant  Value=0
  Constant3 : Constant
  Data Type Conversion1 : DataTypeConversion
  Data Type Conversion2 : DataTypeConversion
  Display : Display
  Relational Operator1 : RelationalOperator  OutDataTypeStr=boolean  RndMeth=Simplest
  Saturation : Saturate  UpperLimit=inf  LowerLimit=2
  Scope : Scope
  Scope1 : Scope
  Scope2 : Scope
  Switch : Switch  Threshold=1
  Unit Delay : UnitDelay  SampleTime=-1  HasFrameUpgradeWarning=on
  Unit Delay1 : UnitDelay  SampleTime=-1  HasFrameUpgradeWarning=on
  Trigger : Outport  VectorParamsAs1DForOutWhenUnconnected=off
  wires:
  Saturation/1 -> Add2/1
  Add/1 -> Switch/1
  In1/1 -> Data Type Conversion2/1
  Unit Delay/1 -> Add/1
  Switch/1 -> Relational Operator1/1, Scope1/1, Unit Delay/1
  Add1/1 -> Scope/1, Unit Delay1/1, Display/1
  Unit Delay1/1 -> Add1/1
  Constant1/1 -> Add1/2
  Relational Operator1/1 -> Scope2/1, Trigger/1
  Data Type Conversion1/1 -> Relational Operator1/2
  Constant2/1 -> Switch/3
  Data Type Conversion2/1 -> Add/2, Switch/2
  Add2/1 -> Data Type Conversion1/1
  In2/1 -> Saturation/1
  Constant3/1 -> Add2/2

== system EPT/Foreground_TimeBase_5ms/E//W /CAN_E//W/CAN_Fault/MCU CAN Fault/deBounce 1/CycleTrigger1 ==
  In1 : Inport
  In2 : Inport  Port=2
  Add : Sum
  Add1 : Sum
  Add2 : Sum  Inputs=+-
  Constant1 : Constant
  Constant2 : Constant  Value=0
  Constant3 : Constant
  Data Type Conversion1 : DataTypeConversion
  Data Type Conversion2 : DataTypeConversion
  Display : Display
  Relational Operator1 : RelationalOperator  OutDataTypeStr=boolean  RndMeth=Simplest
  Saturation : Saturate  UpperLimit=inf  LowerLimit=2
  Scope : Scope
  Scope1 : Scope
  Scope2 : Scope
  Switch : Switch  Threshold=1
  Unit Delay : UnitDelay  SampleTime=-1  HasFrameUpgradeWarning=on
  Unit Delay1 : UnitDelay  SampleTime=-1  HasFrameUpgradeWarning=on
  Trigger : Outport  VectorParamsAs1DForOutWhenUnconnected=off
  wires:
  Constant3/1 -> Add2/2
  In2/1 -> Saturation/1
  Add2/1 -> Data Type Conversion1/1
  Data Type Conversion2/1 -> Switch/2, Add/2
  Constant2/1 -> Switch/3
  Data Type Conversion1/1 -> Relational Operator1/2
  Relational Operator1/1 -> Trigger/1, Scope2/1
  Constant1/1 -> Add1/2
  Unit Delay1/1 -> Add1/1
  Add1/1 -> Display/1, Unit Delay1/1, Scope/1
  Switch/1 -> Unit Delay/1, Scope1/1, Relational Operator1/1
  Unit Delay/1 -> Add/1
  In1/1 -> Data Type Conversion2/1
  Add/1 -> Switch/1
  Saturation/1 -> Add2/1

== system EPT/Foreground_TimeBase_5ms/E//W /CAN_E//W/CAN_Fault/MCU CAN Fault/deBounce 10/CycleTrigger1 ==
  In1 : Inport
  In2 : Inport  Port=2
  Add : Sum
  Add1 : Sum
  Add2 : Sum  Inputs=+-
  Constant1 : Constant
  Constant2 : Constant  Value=0
  Constant3 : Constant
  Data Type Conversion1 : DataTypeConversion
  Data Type Conversion2 : DataTypeConversion
  Display : Display
  Relational Operator1 : RelationalOperator  OutDataTypeStr=boolean  RndMeth=Simplest
  Saturation : Saturate  UpperLimit=inf  LowerLimit=2
  Scope : Scope
  Scope1 : Scope
  Scope2 : Scope
  Switch : Switch  Threshold=1
  Unit Delay : UnitDelay  SampleTime=-1  HasFrameUpgradeWarning=on
  Unit Delay1 : UnitDelay  SampleTime=-1  HasFrameUpgradeWarning=on
  Trigger : Outport  VectorParamsAs1DForOutWhenUnconnected=off
  wires:
  Saturation/1 -> Add2/1
  Add/1 -> Switch/1
  In1/1 -> Data Type Conversion2/1
  Unit Delay/1 -> Add/1
  Switch/1 -> Relational Operator1/1, Scope1/1, Unit Delay/1
  Add1/1 -> Scope/1, Unit Delay1/1, Display/1
  Unit Delay1/1 -> Add1/1
  Constant1/1 -> Add1/2
  Relational Operator1/1 -> Scope2/1, Trigger/1
  Data Type Conversion1/1 -> Relational Operator1/2
  Constant2/1 -> Switch/3
  Data Type Conversion2/1 -> Add/2, Switch/2
  Add2/1 -> Data Type Conversion1/1
  In2/1 -> Saturation/1
  Constant3/1 -> Add2/2

== system EPT/Foreground_TimeBase_5ms/E//W /CAN_E//W/CAN_Fault/MCU CAN Fault/deBounce 2/CycleTrigger1 ==
  In1 : Inport
  In2 : Inport  Port=2
  Add : Sum
  Add1 : Sum
  Add2 : Sum  Inputs=+-
  Constant1 : Constant
  Constant2 : Constant  Value=0
  Constant3 : Constant
  Data Type Conversion1 : DataTypeConversion
  Data Type Conversion2 : DataTypeConversion
  Display : Display
  Relational Operator1 : RelationalOperator  OutDataTypeStr=boolean  RndMeth=Simplest
  Saturation : Saturate  UpperLimit=inf  LowerLimit=2
  Scope : Scope
  Scope1 : Scope
  Scope2 : Scope
  Switch : Switch  Threshold=1
  Unit Delay : UnitDelay  SampleTime=-1  HasFrameUpgradeWarning=on
  Unit Delay1 : UnitDelay  SampleTime=-1  HasFrameUpgradeWarning=on
  Trigger : Outport  VectorParamsAs1DForOutWhenUnconnected=off
  wires:
  Saturation/1 -> Add2/1
  Add/1 -> Switch/1
  In1/1 -> Data Type Conversion2/1
  Unit Delay/1 -> Add/1
  Switch/1 -> Relational Operator1/1, Scope1/1, Unit Delay/1
  Add1/1 -> Scope/1, Unit Delay1/1, Display/1
  Unit Delay1/1 -> Add1/1
  Constant1/1 -> Add1/2
  Relational Operator1/1 -> Scope2/1, Trigger/1
  Data Type Conversion1/1 -> Relational Operator1/2
  Constant2/1 -> Switch/3
  Data Type Conversion2/1 -> Add/2, Switch/2
  Add2/1 -> Data Type Conversion1/1
  In2/1 -> Saturation/1
  Constant3/1 -> Add2/2

== system EPT/Foreground_TimeBase_5ms/E//W /CAN_E//W/CAN_Fault/MCU CAN Fault/deBounce 3/CycleTrigger1 ==
  In1 : Inport
  In2 : Inport  Port=2
  Add : Sum
  Add1 : Sum
  Add2 : Sum  Inputs=+-
  Constant1 : Constant
  Constant2 : Constant  Value=0
  Constant3 : Constant
  Data Type Conversion1 : DataTypeConversion
  Data Type Conversion2 : DataTypeConversion
  Display : Display
  Relational Operator1 : RelationalOperator  OutDataTypeStr=boolean  RndMeth=Simplest
  Saturation : Saturate  UpperLimit=inf  LowerLimit=2
  Scope : Scope
  Scope1 : Scope
  Scope2 : Scope
  Switch : Switch  Threshold=1
  Unit Delay : UnitDelay  SampleTime=-1  HasFrameUpgradeWarning=on
  Unit Delay1 : UnitDelay  SampleTime=-1  HasFrameUpgradeWarning=on
  Trigger : Outport  VectorParamsAs1DForOutWhenUnconnected=off
  wires:
  Constant3/1 -> Add2/2
  In2/1 -> Saturation/1
  Add2/1 -> Data Type Conversion1/1
  Data Type Conversion2/1 -> Switch/2, Add/2
  Constant2/1 -> Switch/3
  Data Type Conversion1/1 -> Relational Operator1/2
  Relational Operator1/1 -> Trigger/1, Scope2/1
  Constant1/1 -> Add1/2
  Unit Delay1/1 -> Add1/1
  Add1/1 -> Display/1, Unit Delay1/1, Scope/1
  Switch/1 -> Unit Delay/1, Scope1/1, Relational Operator1/1
  Unit Delay/1 -> Add/1
  In1/1 -> Data Type Conversion2/1
  Add/1 -> Switch/1
  Saturation/1 -> Add2/1

== system EPT/Foreground_TimeBase_5ms/E//W /CAN_E//W/CAN_Fault/OBC CAN Fault/deBounce 1 /CycleTrigger1 ==
  In1 : Inport
  In2 : Inport  Port=2
  Add : Sum
  Add1 : Sum
  Add2 : Sum  Inputs=+-
  Constant1 : Constant
  Constant2 : Constant  Value=0
  Constant3 : Constant
  Data Type Conversion1 : DataTypeConversion
  Data Type Conversion2 : DataTypeConversion
  Display : Display
  Relational Operator1 : RelationalOperator  OutDataTypeStr=boolean  RndMeth=Simplest
  Saturation : Saturate  UpperLimit=inf  LowerLimit=2
  Scope : Scope
  Scope1 : Scope
  Scope2 : Scope
  Switch : Switch  Threshold=1
  Unit Delay : UnitDelay  SampleTime=-1  HasFrameUpgradeWarning=on
  Unit Delay1 : UnitDelay  SampleTime=-1  HasFrameUpgradeWarning=on
  Trigger : Outport  VectorParamsAs1DForOutWhenUnconnected=off
  wires:
  Saturation/1 -> Add2/1
  Add/1 -> Switch/1
  In1/1 -> Data Type Conversion2/1
  Unit Delay/1 -> Add/1
  Switch/1 -> Relational Operator1/1, Scope1/1, Unit Delay/1
  Add1/1 -> Scope/1, Unit Delay1/1, Display/1
  Unit Delay1/1 -> Add1/1
  Constant1/1 -> Add1/2
  Relational Operator1/1 -> Scope2/1, Trigger/1
  Data Type Conversion1/1 -> Relational Operator1/2
  Constant2/1 -> Switch/3
  Data Type Conversion2/1 -> Add/2, Switch/2
  Add2/1 -> Data Type Conversion1/1
  In2/1 -> Saturation/1
  Constant3/1 -> Add2/2

== system EPT/Foreground_TimeBase_5ms/E//W /CAN_E//W/CAN_Fault/OBC CAN Fault/deBounce 2/CycleTrigger1 ==
  In1 : Inport
  In2 : Inport  Port=2
  Add : Sum
  Add1 : Sum
  Add2 : Sum  Inputs=+-
  Constant1 : Constant
  Constant2 : Constant  Value=0
  Constant3 : Constant
  Data Type Conversion1 : DataTypeConversion
  Data Type Conversion2 : DataTypeConversion
  Display : Display
  Relational Operator1 : RelationalOperator  OutDataTypeStr=boolean  RndMeth=Simplest
  Saturation : Saturate  UpperLimit=inf  LowerLimit=2
  Scope : Scope
  Scope1 : Scope
  Scope2 : Scope
  Switch : Switch  Threshold=1
  Unit Delay : UnitDelay  SampleTime=-1  HasFrameUpgradeWarning=on
  Unit Delay1 : UnitDelay  SampleTime=-1  HasFrameUpgradeWarning=on
  Trigger : Outport  VectorParamsAs1DForOutWhenUnconnected=off
  wires:
  Constant3/1 -> Add2/2
  In2/1 -> Saturation/1
  Add2/1 -> Data Type Conversion1/1
  Data Type Conversion2/1 -> Switch/2, Add/2
  Constant2/1 -> Switch/3
  Data Type Conversion1/1 -> Relational Operator1/2
  Relational Operator1/1 -> Trigger/1, Scope2/1
  Constant1/1 -> Add1/2
  Unit Delay1/1 -> Add1/1
  Add1/1 -> Display/1, Unit Delay1/1, Scope/1
  Switch/1 -> Unit Delay/1, Scope1/1, Relational Operator1/1
  Unit Delay/1 -> Add/1
  In1/1 -> Data Type Conversion2/1
  Add/1 -> Switch/1
  Saturation/1 -> Add2/1

== system EPT/Foreground_TimeBase_5ms/System Setup/HV_Setup()/CHG_Mode/CHG Full Flag/Delay/CycleTrigger ==
  In1 : Inport
  In2 : Inport  Port=2
  Add : Sum
  Add2 : Sum  Inputs=+-
  Constant2 : Constant  Value=0
  Constant3 : Constant
  Data Type Conversion1 : DataTypeConversion
  Data Type Conversion2 : DataTypeConversion
  Relational Operator1 : RelationalOperator  OutDataTypeStr=boolean  RndMeth=Simplest
  Saturation : Saturate  UpperLimit=inf  LowerLimit=2
  Switch : Switch  Threshold=1
  Unit Delay : UnitDelay  SampleTime=-1  HasFrameUpgradeWarning=on
  Trigger : Outport  VectorParamsAs1DForOutWhenUnconnected=off
  wires:
  Constant3/1 -> Add2/2
  In2/1 -> Saturation/1
  Add2/1 -> Data Type Conversion1/1
  Data Type Conversion2/1 -> Switch/2, Add/2
  Constant2/1 -> Switch/3
  Data Type Conversion1/1 -> Relational Operator1/2
  Relational Operator1/1 -> Trigger/1
  Switch/1 -> Unit Delay/1, Relational Operator1/1
  Unit Delay/1 -> Add/1
  In1/1 -> Data Type Conversion2/1
  Add/1 -> Switch/1
  Saturation/1 -> Add2/1

== system EPT/Foreground_TimeBase_5ms/System Setup/HV_Setup()/CHG_Mode/CHG_Mode_Function/CHG_Mode_Function/Cmd_CHG_Current_PID ==
  "Cmd_CHG_Current_PID " : Subsystem
  CountTrigger : Subsystem
  raptor_adjustment2 : Raptor_lib/Data Storage/raptor_adjustment  paramName='CHG_PID_KP_Time'  nameSource=Parameter  initValue=30  dataType=double  storage=Calibration  calDispType=Number  calEnum={'False', 'True'}  calGain=1.0  calOffset=0.0  calMax=inf  calMin=-inf  calFormat='-1'  calUnit=''  calHelp=''  calAccess=1  calFunction=raptor_xcp_function(gcb)  calDispHeaders=off  calColHeaders={'Col1' 'Col2' 'Col3'}  calRowHeaders={'Row1' 'Row2' 'Row3'}
      settings: SourceProductName=Raptor
  wires:
  CountTrigger/1(Tirgger) -> "Cmd_CHG_Current_PID "/Trigger
  raptor_adjustment2/1 -> CountTrigger/1(Counter)

== system EPT/Foreground_TimeBase_5ms/System Setup/HV_Setup()/CHG_Mode/CHG_Mode_Function/CHG_Mode_Function/OBC Work ==
  Constant : Constant  OutDataTypeStr=boolean
  raptor_data_write12 : Raptor_lib/Data Storage/raptor_data_write  dataName='Flag_Charger_Relay_On'  dataShape=Scalar  idxSource=Input Port  idxRow=1  idxCol=1
      settings: SourceProductName=Raptor
  raptor_data_write3 : Raptor_lib/Data Storage/raptor_data_write  dataName='Relay_CHG_OBC'  dataShape=Scalar  idxSource=Input Port  idxRow=1  idxCol=1
      settings: SourceProductName=Raptor
  wires:
  Constant/1 -> raptor_data_write3/1, raptor_data_write12/1

== system EPT/Foreground_TimeBase_5ms/System Setup/HV_Setup()/CHG_Mode/CHG_Mode_Function/Delay/CycleTrigger ==
  In1 : Inport
  In2 : Inport  Port=2
  Add : Sum
  Add2 : Sum  Inputs=+-
  Constant2 : Constant  Value=0
  Constant3 : Constant
  Data Type Conversion1 : DataTypeConversion
  Data Type Conversion2 : DataTypeConversion
  Relational Operator1 : RelationalOperator  OutDataTypeStr=boolean  RndMeth=Simplest
  Saturation : Saturate  UpperLimit=inf  LowerLimit=2
  Switch : Switch  Threshold=1
  Unit Delay : UnitDelay  SampleTime=-1  HasFrameUpgradeWarning=on
  Trigger : Outport  VectorParamsAs1DForOutWhenUnconnected=off
  wires:
  Saturation/1 -> Add2/1
  Add/1 -> Switch/1
  In1/1 -> Data Type Conversion2/1
  Unit Delay/1 -> Add/1
  Switch/1 -> Relational Operator1/1, Unit Delay/1
  Relational Operator1/1 -> Trigger/1
  Data Type Conversion1/1 -> Relational Operator1/2
  Constant2/1 -> Switch/3
  Data Type Conversion2/1 -> Add/2, Switch/2
  Add2/1 -> Data Type Conversion1/1
  In2/1 -> Saturation/1
  Constant3/1 -> Add2/2

== system EPT/Foreground_TimeBase_5ms/System Setup/HV_Setup()/CHG_Mode/Disable_CHG_Mode_Function/Delay/CycleTrigger ==
  In1 : Inport
  In2 : Inport  Port=2
  Add : Sum
  Add2 : Sum  Inputs=+-
  Constant2 : Constant  Value=0
  Constant3 : Constant
  Data Type Conversion1 : DataTypeConversion
  Data Type Conversion2 : DataTypeConversion
  Relational Operator1 : RelationalOperator  OutDataTypeStr=boolean  RndMeth=Simplest
  Saturation : Saturate  UpperLimit=inf  LowerLimit=2
  Switch : Switch  Threshold=1
  Unit Delay : UnitDelay  SampleTime=-1  HasFrameUpgradeWarning=on
  Trigger : Outport  VectorParamsAs1DForOutWhenUnconnected=off
  wires:
  Saturation/1 -> Add2/1
  Add/1 -> Switch/1
  In1/1 -> Data Type Conversion2/1
  Unit Delay/1 -> Add/1
  Switch/1 -> Relational Operator1/1, Unit Delay/1
  Relational Operator1/1 -> Trigger/1
  Data Type Conversion1/1 -> Relational Operator1/2
  Constant2/1 -> Switch/3
  Data Type Conversion2/1 -> Add/2, Switch/2
  Add2/1 -> Data Type Conversion1/1
  In2/1 -> Saturation/1
  Constant3/1 -> Add2/2

== system EPT/Foreground_TimeBase_5ms/System Setup/HV_Setup()/CHG_Mode/Disable_CHG_Mode_Function/Disable_CHG_Mode_Function/Disable_CHG_Mode_Function ==
  Constant : Constant  OutDataTypeStr=uint8
  Constant1 : Constant  Value=0  OutDataTypeStr=uint8
  Constant2 : Constant  Value=0  OutDataTypeStr=double
  Constant3 : Constant  Value=0  OutDataTypeStr=double
  raptor_data_write : Raptor_lib/Data Storage/raptor_data_write  dataName='EPT_OBC_IOUT_CMD'  dataShape=Scalar  idxSource=Input Port  idxRow=1  idxCol=1
      settings: SourceProductName=Raptor
  raptor_data_write1 : Raptor_lib/Data Storage/raptor_data_write  dataName='EPT_OBC_VOUT_CMD'  dataShape=Scalar  idxSource=Input Port  idxRow=1  idxCol=1
      settings: SourceProductName=Raptor
  raptor_data_write2 : Raptor_lib/Data Storage/raptor_data_write  dataName='EPT_OBC_EN'  dataShape=Scalar  idxSource=Input Port  idxRow=1  idxCol=1
      settings: SourceProductName=Raptor
  raptor_data_write3 : Raptor_lib/Data Storage/raptor_data_write  dataName='EPT_OBC_STA'  dataShape=Scalar  idxSource=Input Port  idxRow=1  idxCol=1
      settings: SourceProductName=Raptor
  wires:
  Constant/1 -> raptor_data_write2/1
  Constant1/1 -> raptor_data_write3/1
  Constant2/1 -> raptor_data_write/1
  Constant3/1 -> raptor_data_write1/1
